simulink model "sl_subsys_fcncall3"  (Simulink 7.6)
settings: Solver=FixedStepDiscrete  StartTime=0.0  StopTime=10.0  FixedStep=1  RelTol=1e-3
Description:
  | Data sharing between two function-call subsystems with common initiator example
  | 
  | The Chart is executing the functions, d1=g() and d2=f(), i.e., invoking
  | f() and g() and then later using d1 and d2 computed by g() and f().
  | The functions, f and g, are sharing data via the signal, s (f/Out1 feeds g/In1).
  | Simulink treats the signal, s, as if it were a data store.
  | 
  | In general the inputs to a function-call subsystem must be executed before the
  | function-call initiator (Chart in this case), except when the signal is coming
  | from a block executed by a common function-call initiator. For our example,
  | Chart is a common function-call initiator of both f() and g(). Therefore,
  | the signal, s, below can be thought of as a data store.
settings Model: Creator=The MathWorks Inc.  CovMetricSettings=d  ExtModeAutoUpdateStatusClock=off
settings DataIOCC: SignalLoggingName=logsOut
settings OptimizationCC: BlockReduction=off  BooleanDataType=off  InlineInvariantSignals=on  InitFltsAndDblsToZero=on
settings DebuggingCC: SaveWithParameterizedLinksMsg=none  SignalResolutionControl=TryResolveAllWithWarning  SolverPrmCheckMsg=none  MultiTaskDSMMsg=warning  MultiTaskCondExecSysMsg=none
settings HardwareCC: TargetUnknown=on
settings SFSimCC: SimParseCustomCode=off
settings RTWCC: IncludeERTFirstTime=on
settings CodeAppCC: CustomSymbolStrFcn=$F$N$M
settings GRTTargetCC: TargetFcnLib=ansi_tfl_tmw.mat

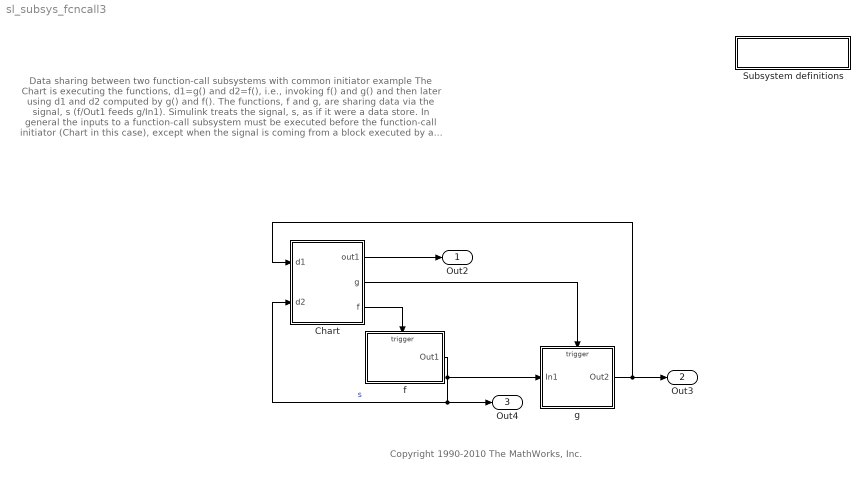
== system sl_subsys_fcncall3 ==
  note: Data sharing between two function-call subsystems with common initiator example
      |
      | The Chart is executing the functions, d1=g() and d2=f(), i.e., invoking
      | f() and g() and then later using d1 and d2 computed by g() and f().
      | The functions, f and g, are sharing data via the signal, s (f/Out1 feeds g/In1).
      | Simulink treats the signal, s, as if it were a data store.
      |
      | In general the inputs to a function-call subsystem must be executed before the
      | function-call initiator (Chart in this case), except when the signal is coming
      | from a block executed by a common function-call initiator. For our example,
      | Chart is a common function-call initiator of both f() and g(). Therefore,
      | the signal, s, below can be thought of as a data store.
  note: Copyright 1990-2010 The MathWorks, Inc.
  " Subsystem definitions" : Subsystem
      settings: OpenFcn=helpview([matlabroot,'/toolbox/simulink/simdemos/simfeatures/html/sl_subsys_definitions.html']);
      mask Display: disp('Subsystem\ndefinitions')
  Chart : Stateflow chart  TreatAsAtomicUnit=on
  f : Subsystem  TreatAsAtomicUnit=on
  g : Subsystem  TreatAsAtomicUnit=on
  Out2 : Outport
  Out3 : Outport  Port=2
  Out4 : Outport  Port=3
  wires:
  Chart/3(f) -> f/Trigger
  f/1(Out1) -> g/1(In1), Out4/1, Chart/2(d2)  "s"
  g/1(Out2) -> Out3/1, Chart/1(d1)
  Chart/1(out1) -> Out2/1
  Chart/2(g) -> g/Trigger

== system sl_subsys_fcncall3/ Subsystem definitions ==

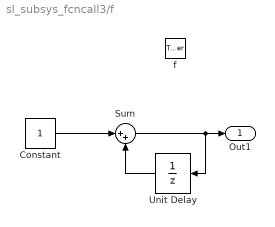
== system sl_subsys_fcncall3/f ==
  f : TriggerPort  TriggerType=function-call  StatesWhenEnabling=reset
  Constant : Constant
  Sum : Sum  Inputs=|++  SaturateOnIntegerOverflow=on  InputSameDT=on  OutDataTypeStr=Inherit: Same as first input
  Unit Delay : UnitDelay  SampleTime=-1
  Out1 : Outport
  wires:
  Constant/1 -> Sum/1
  Unit Delay/1 -> Sum/2
  Sum/1 -> Out1/1, Unit Delay/1

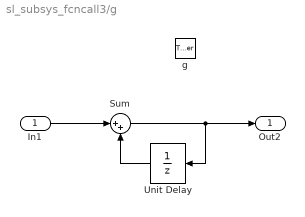
== system sl_subsys_fcncall3/g ==
  In1 : Inport
  g : TriggerPort  TriggerType=function-call  StatesWhenEnabling=reset
  Sum : Sum  Inputs=|++  SaturateOnIntegerOverflow=on  InputSameDT=on  OutDataTypeStr=Inherit: Same as first input
  Unit Delay : UnitDelay  SampleTime=-1
  Out2 : Outport
  wires:
  In1/1 -> Sum/1
  Unit Delay/1 -> Sum/2
  Sum/1 -> Out2/1, Unit Delay/1

== stateflow chart Chart ==
  state one/
    entry: g; out1= d1+d2;
  state two/
    entry: f; out1=d1-d2;
  one -> two
  two -> one
  (default) -> one
  data: d1 input double; d2 input double; out1 output double
  events: g output FUNCTION_CALL_EVENT; f output FUNCTION_CALL_EVENT
